simulink model "demux1to2"  (R2020a)
settings: Solver=VariableStepAuto  StartTime=0.0  StopTime=10.0  RelTol=1e-3
settings Model: Creator=kishan  LastModifiedBy=kishan

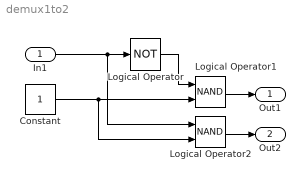
== system demux1to2 ==
  In1 : Inport
  Constant : Constant
  Logical Operator : Logic  Operator=NOT  AllPortsSameDT=off  OutDataTypeStr=boolean
  Logical Operator1 : Logic  Operator=NAND  AllPortsSameDT=off  OutDataTypeStr=boolean
  Logical Operator2 : Logic  Operator=NAND  AllPortsSameDT=off  OutDataTypeStr=boolean
  Out1 : Outport
  Out2 : Outport  Port=2
  wires:
  Logical Operator/1 -> Logical Operator1/1
  In1/1 -> Logical Operator2/1, Logical Operator/1
  Constant/1 -> Logical Operator2/2, Logical Operator1/2
  Logical Operator1/1 -> Out1/1
  Logical Operator2/1 -> Out2/1
